simulink model "sistema"  (R2025b)
settings: Solver=ode23t  StartTime=0.0  StopTime=10.0  MaxStep=0.001  RelTol=1e-3
libraries: slpidlib x1, simulink x1
settings DataIOCC: ReturnWorkspaceOutputs=off  TimeSaveName=t
settings DebuggingCC: AlgebraicLoopMsg=none  ArtificialAlgebraicLoopMsg=none  MaxConsecutiveZCsMsg=none

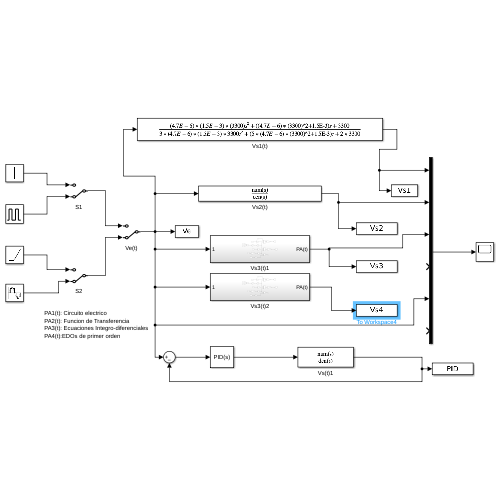
[thumbnail: Simulink's stored preview of the top-level diagram]
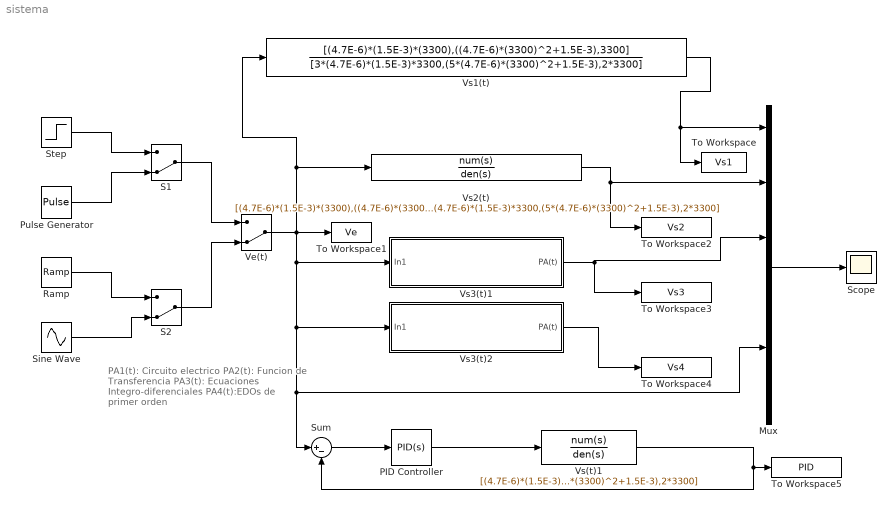
== system sistema ==
  note: PA1(t): Circuito electrico
      | PA2(t): Funcion de Transferencia
      | PA3(t): Ecuaciones Integro-diferenciales
      | PA4(t):EDOs de primer orden
  Mux : Mux  Inputs=6
  PID Controller : slpidlib/PID Controller  Controller=PID  Form=Parallel  TimeDomain=Continuous-time  UseExternalTs=off  SampleTime=-1  IntegratorMethod=Forward Euler  FilterMethod=Forward Euler  ControllerParametersSource=internal  P=0  I=699636.30057331  UseKiTs=off  D=0  UseExternalDerivativeSource=off  N=100  UseFilter=on  TunerSelectOption=Transfer Function Based (PID Tuner App)  InitialConditionSource=internal  InitialConditionForIntegrator=0  InitialConditionForFilter=0  DifferentiatorICPrevScaledInput=0  ExternalReset=none  TrackingMode=off  Kt=1  LimitOutput=off  SatLimitsSource=internal  UpperSaturationLimit=inf  LowerSaturationLimit=-inf  LinearizeAsGain=on  AntiWindupMode=none  Kb=1  LimitIntegrator=off  UpperIntegratorSaturationLimit=inf  LowerIntegratorSaturationLimit=-inf  POutMin=[]  POutMax=[]  IOutMin=[]  IOutMax=[]  DOutMin=[]  DOutMax=[]  NOutMin=[]  NOutMax=[]  SumOutMin=[]  SumOutMax=[]  SaturationOutMin=[]  SaturationOutMax=[]  PParamMin=[]  PParamMax=[]  IParamMin=[]  IParamMax=[]  DParamMin=[]  DParamMax=[]  NParamMin=[]  NParamMax=[]  KbParamMin=[]  KbParamMax=[]  KtParamMin=[]  KtParamMax=[]  KbOutMin=[]  KbOutMax=[]  KtOutMin=[]  KtOutMax=[]  IntegratorOutMin=[]  IntegratorOutMax=[]  FilterOutMin=[]  FilterOutMax=[]  SumI1OutMin=[]  SumI1OutMax=[]  SumI2OutMin=[]  SumI2OutMax=[]  SumI3OutMin=[]  SumI3OutMax=[]  SumI4OutMin=[]  SumI4OutMax=[]  SumDOutMin=[]  SumDOutMax=[]  DifferentiatorOutMin=[]  DifferentiatorOutMax=[]  FilterDiffOutCoefMin=[]  FilterDiffOutCoefMax=[]  ReciprocalOutMin=[]  ReciprocalOutMax=[]  SumDenOutMin=[]  SumDenOutMax=[]  SumNumOutMin=[]  SumNumOutMax=[]  DivideOutMin=[]  DivideOutMax=[]  UdiffTsProdOutMin=[]  UdiffTsProdOutMax=[]  NTsProdOutMin=[]  NTsProdOutMax=[]  UintegralTsProdOutMin=[]  UintegralTsProdOutMax=[]  UngainTsProdOutMin=[]  UngainTsProdOutMax=[]  ClampingZeroOutDataTypeStr=Inherit: Inherit via back propagation  ClampingZeroOutMin=[]  ClampingZeroOutMax=[]  FilterDenConstantOutDataTypeStr=Inherit: Inherit via back propagation  FilterDenConstantOutMin=[]  FilterDenConstantOutMax=[]  PCopyOutDataTypeStr=Inherit: Inherit via back propagation  PCopyOutMin=[]  PCopyOutMax=[]  NCopyOutDataTypeStr=Inherit: Inherit via back propagation  NCopyOutMin=[]  NCopyOutMax=[]  IntegratorContinuousStateAttributes=''  IntegratorStateMustResolveToSignalObject=off  IntegratorRTWStateStorageClass=Auto  FilterContinuousStateAttributes=''  FilterStateMustResolveToSignalObject=off  FilterRTWStateStorageClass=Auto  ParallelPVariant=InternalParameters  IdealPVariant=Disabled  IVariant=InternalParameters  DVariant=InternalParameters  IntegratorVariant=Continuous  SatVariant=Disabled  AWVariant=Passthrough  PCopyVariant=Disabled  TRVariant=Disabled  FdbkBlocksVariant=Forward  IdealPFdbkVariant=Disabled  SatFdbkVariant=Disabled  DerivativeFilterVariant=ContFilter  NVariant=InternalParameters  NCopyVariant=Disabled  FilterICVariant=InternalICsFilter  IntegratorICVariant=InternalICs  ExternalResetVariant=Disabled  TRSumVariant=Passthrough  SumFdbkVariant=Disabled  SumVariant=Sum_PID  TsampFilterVariant=InternalTs  TsampNgainVariant=Passthrough  TsampIntegralVariant=Disabled_SignalSpec  ExternalSaturationOutDataTypeStr=Inherit: Same as second input  DerivativeSourceVariant=ErrorSignal  PreIntVariant=InternalPreInt
  Pulse Generator : DiscretePulseGenerator  PulseType=Time based  Period=10  PulseWidth=10  PhaseDelay=1
  Ramp : simulink/Sources/Ramp  slope=1/10  start=0  InitialOutput=0
  S1 : ManualSwitch  CurrentSetting=0
  S2 : ManualSwitch  CurrentSetting=0
  Scope : Scope
      settings: ActiveDisplayYMinimum=0.031018066614822426  ActiveDisplayYMaximum=1.0008673605640266
  Sine Wave : Sin  Frequency=pi/2  SampleTime=0.01
  Step : Step  Time=0  SampleTime=0.001
  Sum : Sum  Inputs=|+-
  To Workspace : ToWorkspace  VariableName=Vs1  SampleTime=-1
  To Workspace1 : ToWorkspace  VariableName=Ve  SampleTime=-1
  To Workspace2 : ToWorkspace  VariableName=Vs2  SampleTime=-1
  To Workspace3 : ToWorkspace  VariableName=Vs3  SampleTime=-1
  To Workspace4 : ToWorkspace  VariableName=Vs4  SampleTime=-1
  To Workspace5 : ToWorkspace  VariableName=PID  SampleTime=-1
  Ve(t) : ManualSwitch  CurrentSetting=0
  Vs(t)1 : TransferFcn  Numerator=[(4.7E-6)*(1.5E-3)*(3300),((4.7E-6)*(3300)^2+1.5E-3),3300]  Denominator=[3*(4.7E-6)*(1.5E-3)*3300,(5*(4.7E-6)*(3300)^2+1.5E-3),2*3300]
  Vs1(t) : TransferFcn  Numerator=[(4.7E-6)*(1.5E-3)*(3300),((4.7E-6)*(3300)^2+1.5E-3),3300]  Denominator=[3*(4.7E-6)*(1.5E-3)*3300,(5*(4.7E-6)*(3300)^2+1.5E-3),2*3300]
  Vs2(t) : TransferFcn  Numerator=[(4.7E-6)*(1.5E-3)*(3300),((4.7E-6)*(3300)^2+1.5E-3),3300]  Denominator=[3*(4.7E-6)*(1.5E-3)*3300,(5*(4.7E-6)*(3300)^2+1.5E-3),2*3300]
  Vs3(t)1 : Subsystem
  Vs3(t)2 : Subsystem
  wires:
  Step/1 -> S1/1
  Pulse Generator/1 -> S1/2
  Ramp/1 -> S2/1
  Sine Wave/1 -> S2/2
  S2/1 -> Ve(t)/2
  S1/1 -> Ve(t)/1
  Ve(t)/1 -> To Workspace1/1, Vs3(t)1/1(In1), Vs3(t)2/1(In1), Sum/1, Mux/5, Vs1(t)/1, Vs2(t)/1
  Vs3(t)2/1(PA(t)) -> To Workspace4/1
  Vs2(t)/1 -> Mux/2, To Workspace2/1
  Vs3(t)1/1(PA(t)) -> To Workspace3/1, Mux/3
  Mux/1 -> Scope/1
  Vs1(t)/1 -> To Workspace/1, Mux/1
  Sum/1 -> PID Controller/1
  PID Controller/1 -> Vs(t)1/1
  Vs(t)1/1 -> To Workspace5/1, Sum/2

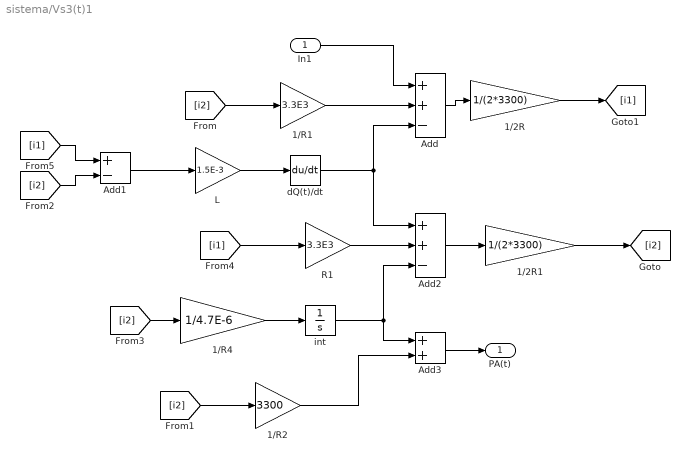
== system sistema/Vs3(t)1 ==
  In1 : Inport
  1/2R : Gain  Gain=1/(2*3300)
  1/2R1 : Gain  Gain=1/(2*3300)
  1/R1 : Gain  Gain=3.3E3
  1/R2 : Gain  Gain=3300
  1/R4 : Gain  Gain=1/4.7E-6
  Add : Sum  Inputs=++-
  Add1 : Sum  Inputs=+-
  Add2 : Sum  Inputs=++-
  Add3 : Sum
  L : Gain  Gain=1.5E-3
  R1 : Gain  Gain=3.3E3
  dQ(t)/dt : Derivative
  int : Integrator
  PA(t) : Outport
  wires:
  In1/1 -> Add/1
  Add/1 -> 1/2R/1
  [i2] -> 1/R1/1
  dQ(t)/dt/1 -> Add2/1, Add/3
  1/R1/1 -> Add/2
  [i1] -> Add1/1
  [i2] -> Add1/2
  Add1/1 -> L/1
  L/1 -> dQ(t)/dt/1
  [i1] -> R1/1
  R1/1 -> Add2/2
  int/1 -> Add3/1, Add2/3
  Add3/1 -> PA(t)/1
  Add2/1 -> 1/2R1/1
  1/2R1/1 -> [i2]
  1/2R/1 -> [i1]
  [i2] -> 1/R4/1
  1/R4/1 -> int/1
  [i2] -> 1/R2/1
  1/R2/1 -> Add3/2

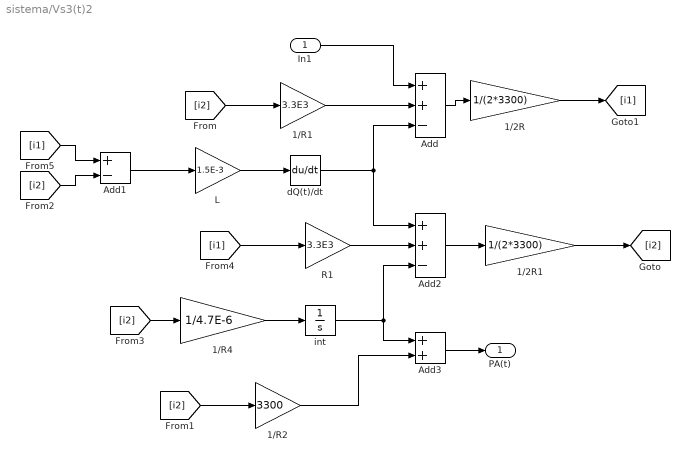
== system sistema/Vs3(t)2 ==
  In1 : Inport
  1/2R : Gain  Gain=1/(2*3300)
  1/2R1 : Gain  Gain=1/(2*3300)
  1/R1 : Gain  Gain=3.3E3
  1/R2 : Gain  Gain=3300
  1/R4 : Gain  Gain=1/4.7E-6
  Add : Sum  Inputs=++-
  Add1 : Sum  Inputs=+-
  Add2 : Sum  Inputs=++-
  Add3 : Sum
  L : Gain  Gain=1.5E-3
  R1 : Gain  Gain=3.3E3
  dQ(t)/dt : Derivative
  int : Integrator
  PA(t) : Outport
  wires:
  1/R2/1 -> Add3/2
  [i2] -> 1/R2/1
  1/R4/1 -> int/1
  [i2] -> 1/R4/1
  1/2R/1 -> [i1]
  1/2R1/1 -> [i2]
  Add2/1 -> 1/2R1/1
  Add3/1 -> PA(t)/1
  int/1 -> Add2/3, Add3/1
  R1/1 -> Add2/2
  [i1] -> R1/1
  L/1 -> dQ(t)/dt/1
  Add1/1 -> L/1
  [i2] -> Add1/2
  [i1] -> Add1/1
  1/R1/1 -> Add/2
  dQ(t)/dt/1 -> Add/3, Add2/1
  [i2] -> 1/R1/1
  Add/1 -> 1/2R/1
  In1/1 -> Add/1
